simulink library "vmc"  (R2021b)
settings: Solver=VariableStepAuto  StartTime=0.0  StopTime=10.0  RelTol=1e-3
undefined symbols (not defined in the file or in its folder): AVMC_ACCDeltaTqIGain_X_kph, AVMC_ACCDeltaTqIGain_Y_mps2, AVMC_ACCDeltaTqIGainP2_X_kph, AVMC_ACCDeltaTqIGainP2_Y_mps2, AVMC_ACCDeltaTqPGain_X_kph, AVMC_ACCDeltaTqPGain_Y_kph, AVMC_ACCDeltaTqPGainP2_X_kph, AVMC_ACCDeltaTqPGainP2_Y_kph, AVMC_ACCLongSteadyCtrl_X_kph, AVMC_CCAccelCMD_X_kph, AVMC_CCAccelCMD_Y_kph, AVMC_CCDeltaTqIGain_X_kph, AVMC_CCDeltaTqIGain_Y_mps2, AVMC_CCDeltaTqPGain_X_kph, AVMC_CCDeltaTqPGain_Y_kph, AVMC_CCLongSteadyCtrl_X_kph, AVMC_DISCDeltaTqIGainP2_X_kph, AVMC_DISCDeltaTqIGainP2_Y_mps2, AVMC_ESCRegenOut_X_kph, AVMC_ESCRegenOut_Y_Deg, AVMC_ESCRegenOutEnSpd_X_Deg, AVMC_LatESCRegenOut_X_kph, AVMC_LatESCRegenOut_Y_Deg, AVMC_LongAccDeadZone_X_kph, AVMC_LongAccDeadZoneP2_X_kph, AVMC_LongAccFiltTs_X_Gps, AVMC_LongAccFiltTsP2_X_Gps, AVMC_MCPresBaseTq_X_bar, AVMC_MSAAccelCMD_X_kph, AVMC_MSAAccelCMD_Y_kph, AVMC_MSADeltaTqIGain_X_kph, AVMC_MSADeltaTqIGain_Y_mps2, AVMC_MSADeltaTqPGain_X_kph, AVMC_MSADeltaTqPGain_Y_kph, AVMC_MSALongSteadyCtrl_X_kph, AVMC_MSAPedalOvrd_X_kph, AVMC_MSASpdBand_X_kph, AVMC_OPDDisSlideRate_X_Deg, AVMC_RDCDetectTime_X_kph, AVMC_RDCDetectTime_Y_pct, AVMC_RDCEnSlideRate_X_Deg, AVMC_StESCYaw_X_kph, AVMC_StESCYaw_Y_Deg, AVMC_StESCYawCom_X_kph, AVMC_StESCYawCom_Y_Gps, AVMC_TMSpdBaseTq_X_rpm, C_TASK_10MS_S, C_TASK_5MS_S, DEG2RAD, Discrete, ENUM_ADASACCSTA_ACTIVE, ENUM_ADASACCSTA_OVERRIDE, ENUM_ADASACCSTA_STANDBY, ENUM_ADASMSASTA_ACTIVE, ENUM_ADASMSASTA_ERROR, ENUM_ADASMSASTA_OFF, ENUM_ADASMSASTA_OVERSPEED, ENUM_ADASMSASTA_STANDBY, ENUM_ADASMSASTA_UNDERSPEED, ENUM_ADASMSASTA_UNLIMIT ... (+254)
libraries: hcu_lib x57, simulink x49, ctrlSharedLib x6, simulink_extras x1
(part 3 of 9)

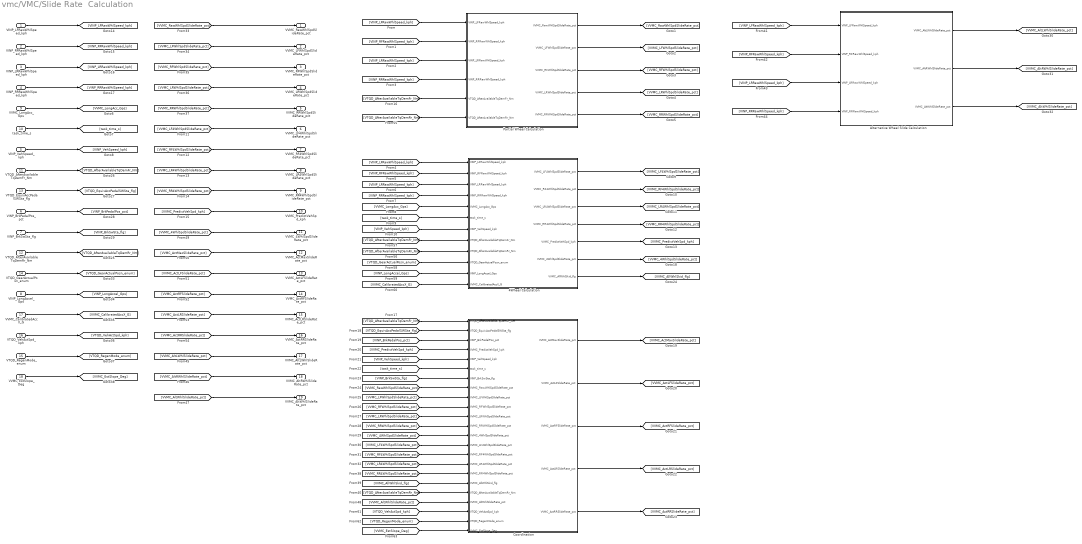
== system vmc/VMC/Slide Rate  Calculation ==
  VINP_LFRawWhlSpeed_kph : Inport
  VINP_RFRawWhlSpeed_kph : Inport  Port=2
  VINP_LRRawWhlSpeed_kph : Inport  Port=3
  VINP_RRRawWhlSpeed_kph : Inport  Port=4
  VINP_VehSpeed_kph : Inport  Port=5
  VINP_BrkPedalPos_pct : Inport  Port=6
  VINP_BrkSwSta_flg : Inport  Port=7
  VINP_LongAccel_Gps : Inport  Port=8
  VVMC_LongAcc_Gps : Inport  Port=9
  task_time_s : Inport  Port=10
  VTQD_AfterAvailableTqDemFr_Nm : Inport  Port=11
  VTQD_AfterAvailableTqDemRr_Nm : Inport  Port=12
  VTQD_EquivAccPedalSWSta_flg : Inport  Port=13
  VTQD_GearActualPosn_enum : Inport  Port=14
  VTQD_RegenMode_enum : Inport  Port=15
  VTQD_VehActSpd_kph : Inport  Port=16
  VVMC_CalibratedAccX_G : Inport  Port=17
  VVMC_EstSlope_Deg : Inport  Port=18
  4Wheel Calculation : Subsystem
  Alternative Wheel Slide Calculation : Subsystem
  Coordination : Subsystem
  Partial Wheel Calculation : Subsystem
  VVMC_RawWhlSpdSlideRate_pct : Outport
  VVMC_LFWhlSpdSlideRate_pct : Outport  Port=2
  VVMC_RFWhlSpdSlideRate_pct : Outport  Port=3
  VVMC_LRWhlSpdSlideRate_pct : Outport  Port=4
  VVMC_RRWhlSpdSlideRate_pct : Outport  Port=5
  VVMC_LF4WhlSpdSlideRate_pct : Outport  Port=6
  VVMC_RF4WhlSpdSlideRate_pct : Outport  Port=7
  VVMC_LR4WhlSpdSlideRate_pct : Outport  Port=8
  VVMC_RR4WhlSpdSlideRate_pct : Outport  Port=9
  VVMC_PredictVehSpd_kph : Outport  Port=10
  VVMC_4WhlSpdSlideRate_pct : Outport  Port=11
  VVMC_ActMaxSlideRate_pct : Outport  Port=12
  VVMC_ActLFSlideRate_pct : Outport  Port=13
  VVMC_ActRFSlideRate_pct : Outport  Port=14
  VVMC_ActLRSlideRate_pct : Outport  Port=15
  VVMC_ActRRSlideRate_pct : Outport  Port=16
  VVMC_AltLWhlSlideRate_pct : Outport  Port=17
  VVMC_AltRWhlSlideRate_pct : Outport  Port=18
  VVMC_AltWhlSlideRate_pct : Outport  Port=19
  wires:
  VINP_BrkSwSta_flg/1 -> [VINP_BrkSwSta_flg]
  VTQD_AfterAvailableTqDemFr_Nm/1 -> [VTQD_AfterAvailableTqDemFr_Nm]
  [VVMC_RF4WhlSpdSlideRate_pct] -> VVMC_RF4WhlSpdSlideRate_pct/1
  [VVMC_ActRRSlideRate_pct] -> VVMC_ActRRSlideRate_pct/1
  VTQD_EquivAccPedalSWSta_flg/1 -> [VTQD_EquivAccPedalSWSta_flg]
  [VVMC_LFWhlSpdSlideRate_pct] -> VVMC_LFWhlSpdSlideRate_pct/1
  VINP_BrkPedalPos_pct/1 -> [VINP_BrkPedalPos_pct]
  [VVMC_RRWhlSpdSlideRate_pct] -> VVMC_RRWhlSpdSlideRate_pct/1
  task_time_s/1 -> [task_time_s]
  VINP_RRRawWhlSpeed_kph/1 -> [VINP_RRRawWhlSpeed_kph]
  [VVMC_ActMaxSlideRate_pct] -> VVMC_ActMaxSlideRate_pct/1
  [VVMC_RFWhlSpdSlideRate_pct] -> VVMC_RFWhlSpdSlideRate_pct/1
  [VVMC_LR4WhlSpdSlideRate_pct] -> VVMC_LR4WhlSpdSlideRate_pct/1
  [VVMC_ActRFSlideRate_pct] -> VVMC_ActRFSlideRate_pct/1
  [VVMC_RR4WhlSpdSlideRate_pct] -> VVMC_RR4WhlSpdSlideRate_pct/1
  VINP_RFRawWhlSpeed_kph/1 -> [VINP_RFRawWhlSpeed_kph]
  VINP_VehSpeed_kph/1 -> [VINP_VehSpeed_kph]
  [VVMC_ActLRSlideRate_pct] -> VVMC_ActLRSlideRate_pct/1
  [VVMC_PredictVehSpd_kph] -> VVMC_PredictVehSpd_kph/1
  VINP_LRRawWhlSpeed_kph/1 -> [VINP_LRRawWhlSpeed_kph]
  [VVMC_LF4WhlSpdSlideRate_pct] -> VVMC_LF4WhlSpdSlideRate_pct/1
  [VVMC_RawWhlSpdSlideRate_pct] -> VVMC_RawWhlSpdSlideRate_pct/1
  VINP_LFRawWhlSpeed_kph/1 -> [VINP_LFRawWhlSpeed_kph]
  [VVMC_LRWhlSpdSlideRate_pct] -> VVMC_LRWhlSpdSlideRate_pct/1
  [VVMC_ActLFSlideRate_pct] -> VVMC_ActLFSlideRate_pct/1
  [VVMC_4WhlSpdSlideRate_pct] -> VVMC_4WhlSpdSlideRate_pct/1
  VVMC_LongAcc_Gps/1 -> [VVMC_LongAcc_Gps]
  VTQD_AfterAvailableTqDemRr_Nm/1 -> [VTQD_AfterAvailableTqDemRr_Nm]
  [VINP_LFRawWhlSpeed_kph] -> Alternative Wheel Slide Calculation/1(VINP_LFRawWhlSpeed_kph)
  [VINP_RFRawWhlSpeed_kph] -> Alternative Wheel Slide Calculation/2(VINP_RFRawWhlSpeed_kph)
  [VINP_LRRawWhlSpeed_kph] -> Alternative Wheel Slide Calculation/3(VINP_LRRawWhlSpeed_kph)
  [VINP_RRRawWhlSpeed_kph] -> Alternative Wheel Slide Calculation/4(VINP_RRRawWhlSpeed_kph)
  Alternative Wheel Slide Calculation/1(VVMC_AltLWhlSlideRate_pct) -> [VVMC_AltLWhlSlideRate_pct]
  Alternative Wheel Slide Calculation/2(VVMC_AltRWhlSlideRate_pct) -> [VVMC_AltRWhlSlideRate_pct]
  Alternative Wheel Slide Calculation/3(VVMC_AltWhlSlideRate_pct) -> [VVMC_AltWhlSlideRate_pct]
  [VVMC_AltLWhlSlideRate_pct] -> VVMC_AltLWhlSlideRate_pct/1
  [VVMC_AltRWhlSlideRate_pct] -> VVMC_AltRWhlSlideRate_pct/1
  [VVMC_AltWhlSlideRate_pct] -> VVMC_AltWhlSlideRate_pct/1
  Partial Wheel Calculation/2(VVMC_LFWhlSpdSlideRate_pct) -> [VVMC_LFWhlSpdSlideRate_pct]
  Partial Wheel Calculation/5(VVMC_RRWhlSpdSlideRate_pct) -> [VVMC_RRWhlSpdSlideRate_pct]
  Partial Wheel Calculation/3(VVMC_RFWhlSpdSlideRate_pct) -> [VVMC_RFWhlSpdSlideRate_pct]
  Partial Wheel Calculation/1(VVMC_RawWhlSpdSlideRate_pct) -> [VVMC_RawWhlSpdSlideRate_pct]
  [VINP_RFRawWhlSpeed_kph] -> Partial Wheel Calculation/2(VINP_RFRawWhlSpeed_kph)
  [VINP_LRRawWhlSpeed_kph] -> Partial Wheel Calculation/3(VINP_LRRawWhlSpeed_kph)
  [VTQD_AfterAvailableTqDemFr_Nm] -> Partial Wheel Calculation/5(VTQD_AfterAvailableTqDemFr_Nm)
  [VINP_LFRawWhlSpeed_kph] -> Partial Wheel Calculation/1(VINP_LFRawWhlSpeed_kph)
  [VINP_RRRawWhlSpeed_kph] -> Partial Wheel Calculation/4(VINP_RRRawWhlSpeed_kph)
  [VTQD_AfterAvailableTqDemRr_Nm] -> Partial Wheel Calculation/6(VTQD_AfterAvailableTqDemRr_Nm)
  Partial Wheel Calculation/4(VVMC_LRWhlSpdSlideRate_pct) -> [VVMC_LRWhlSpdSlideRate_pct]
  4Wheel Calculation/3(VVMC_LR4WhlSpdSlideRate_pct) -> [VVMC_LR4WhlSpdSlideRate_pct]
  [task_time_s] -> 4Wheel Calculation/6(task_time_s)
  4Wheel Calculation/1(VVMC_LF4WhlSpdSlideRate_pct) -> [VVMC_LF4WhlSpdSlideRate_pct]
  4Wheel Calculation/7(VVMC_AllWhlSkid_flg) -> [VVMC_AllWhlSkid_flg]
  [VVMC_LongAcc_Gps] -> 4Wheel Calculation/5(VVMC_LongAcc_Gps)
  4Wheel Calculation/4(VVMC_RR4WhlSpdSlideRate_pct) -> [VVMC_RR4WhlSpdSlideRate_pct]
  [VTQD_AfterAvailableTqDemRr_Nm] -> 4Wheel Calculation/9(VTQD_AfterAvailableTqDemRr_Nm)
  [VTQD_AfterAvailableTqDemFr_Nm] -> 4Wheel Calculation/8(VTQD_AfterAvailableTqDemFr_Nm)
  [VINP_VehSpeed_kph] -> 4Wheel Calculation/7(VINP_VehSpeed_kph)
  4Wheel Calculation/5(VVMC_PredictVehSpd_kph) -> [VVMC_PredictVehSpd_kph]
  [VINP_LRRawWhlSpeed_kph] -> 4Wheel Calculation/3(VINP_LRRawWhlSpeed_kph)
  [VINP_RRRawWhlSpeed_kph] -> 4Wheel Calculation/4(VINP_RRRawWhlSpeed_kph)
  [VINP_LFRawWhlSpeed_kph] -> 4Wheel Calculation/1(VINP_LFRawWhlSpeed_kph)
  [VINP_RFRawWhlSpeed_kph] -> 4Wheel Calculation/2(VINP_RFRawWhlSpeed_kph)
  4Wheel Calculation/2(VVMC_RF4WhlSpdSlideRate_pct) -> [VVMC_RF4WhlSpdSlideRate_pct]
  4Wheel Calculation/6(VVMC_4WhlSpdSlideRate_pct) -> [VVMC_4WhlSpdSlideRate_pct]
  [VVMC_LF4WhlSpdSlideRate_pct] -> Coordination/14(VVMC_LF4WhlSpdSlideRate_pct)
  [VVMC_RR4WhlSpdSlideRate_pct] -> Coordination/17(VVMC_RR4WhlSpdSlideRate_pct)
  [VVMC_LR4WhlSpdSlideRate_pct] -> Coordination/16(VVMC_LR4WhlSpdSlideRate_pct)
  [task_time_s] -> Coordination/6(task_time_s)
  [VVMC_LFWhlSpdSlideRate_pct] -> Coordination/9(VVMC_LFWhlSpdSlideRate_pct)
  [VTQD_AfterAvailableTqDemFr_Nm] -> Coordination/1(VTQD_AfterAvailableTqDemFr_Nm)
  [VVMC_AltWhlSlideRate_pct] -> Coordination/20(VVMC_AltWhlSlideRate_pct)
  [VVMC_RFWhlSpdSlideRate_pct] -> Coordination/10(VVMC_RFWhlSpdSlideRate_pct)
  [VTQD_EquivAccPedalSWSta_flg] -> Coordination/2(VTQD_EquivAccPedalSWSta_flg)
  [VVMC_AllWhlSkid_flg] -> Coordination/18(VVMC_AllWhlSkid_flg)
  [VVMC_4WhlSpdSlideRate_pct] -> Coordination/13(VVMC_4WhlSpdSlideRate_pct)
  [VINP_VehSpeed_kph] -> Coordination/5(VINP_VehSpeed_kph)
  Coordination/3(VVMC_ActRFSlideRate_pct) -> [VVMC_ActRFSlideRate_pct]
  [VVMC_RawWhlSpdSlideRate_pct] -> Coordination/8(VVMC_RawWhlSpdSlideRate_pct)
  [VTQD_AfterAvailableTqDemRr_Nm] -> Coordination/19(VTQD_AfterAvailableTqDemRr_Nm)
  Coordination/4(VVMC_ActLRSlideRate_pct) -> [VVMC_ActLRSlideRate_pct]
  [VVMC_PredictVehSpd_kph] -> Coordination/4(VVMC_PredictVehSpd_kph)
  [VINP_BrkSwSta_flg] -> Coordination/7(VINP_BrkSwSta_flg)
  [VVMC_LRWhlSpdSlideRate_pct] -> Coordination/11(VVMC_LRWhlSpdSlideRate_pct)
  [VVMC_RRWhlSpdSlideRate_pct] -> Coordination/12(VVMC_RRWhlSpdSlideRate_pct)
  [VINP_BrkPedalPos_pct] -> Coordination/3(VINP_BrkPedalPos_pct)
  Coordination/1(VVMC_ActMaxSlideRate_pct) -> [VVMC_ActMaxSlideRate_pct]
  Coordination/5(VVMC_ActRRSlideRate_pct) -> [VVMC_ActRRSlideRate_pct]
  Coordination/2(VVMC_ActLFSlideRate_pct) -> [VVMC_ActLFSlideRate_pct]
  [VVMC_RF4WhlSpdSlideRate_pct] -> Coordination/15(VVMC_RF4WhlSpdSlideRate_pct)
  [VTQD_GearActualPosn_enum] -> 4Wheel Calculation/10(VTQD_GearActualPosn_enum)
  VTQD_GearActualPosn_enum/1 -> [VTQD_GearActualPosn_enum]
  VINP_LongAccel_Gps/1 -> [VINP_LongAccel_Gps]
  [VINP_LongAccel_Gps] -> 4Wheel Calculation/11(VINP_LongAccel_Gps)
  [VVMC_CalibratedAccX_G] -> 4Wheel Calculation/12(VVMC_CalibratedAccX_G)
  VVMC_CalibratedAccX_G/1 -> [VVMC_CalibratedAccX_G]
  VVMC_EstSlope_Deg/1 -> [VVMC_EstSlope_Deg]
  VTQD_RegenMode_enum/1 -> [VTQD_RegenMode_enum]
  VTQD_VehActSpd_kph/1 -> [VTQD_VehActSpd_kph]
  [VTQD_RegenMode_enum] -> Coordination/22(VTQD_RegenMode_enum)
  [VTQD_VehActSpd_kph] -> Coordination/21(VTQD_VehActSpd_kph)
  [VVMC_EstSlope_Deg] -> Coordination/23(VVMC_EstSlope_Deg)

== system vmc/VMC/Subsystem1 ==
  note: TRUE
  VINP_VehSpeed_kph : Inport
  VINP_ACCRequiredAccel_mps2 : Inport  Port=2
  VINP_ACCVehHoldReq_flg : Inport  Port=3
  VINP_ACCObjRelSpd_mps : Inport  Port=4
  VINP_ACCObjDist_m : Inport  Port=5
  VINP_TimeGapLevel_enum : Inport  Port=6
  VTQD_FrEDUAvailBrkRgnTq_Nm : Inport  Port=7
  VTQD_RrEDUAvailBrkRgnTq_Nm : Inport  Port=8
  VINP_METERKPHCalcu_kph : Inport  Port=9
  0 : Constant  Value=KVMC_AllowSetSpdOvrd_flg
  1 : Constant  Value=KVMC_AllowSetSpdOvrdVal_flg
  10kph1 : Constant  Value=KVMC_AllowSetSpdSpd_kph
  20m : Constant  Value=KVMC_AllowSetSpdDist_m
  2m : Constant  Value=KVMC_NotAllowSetSpdDist_m
  AND : Logic  AllPortsSameDT=off  OutDataTypeStr=boolean
  AND2 : Logic  Inputs=3  AllPortsSameDT=off  OutDataTypeStr=boolean
  Add : Sum
  Cast To Single : DataTypeConversion  OutDataTypeStr=single
  Constant1 : Constant  Value=KPH2MPS
  Constant10 : Constant  Value=ENUM_TIMEGAPLEVEL_LEVEL1
  Constant11 : Constant  Value=ENUM_TIMEGAPLEVEL_LEVEL2
  Constant12 : Constant  Value=ENUM_TIMEGAPLEVEL_LEVEL3
  Constant13 : Constant  Value=ENUM_TIMEGAPLEVEL_LEVEL4
  Constant14 : Constant  Value=KVMC_TimeGapBandLv2_s
  Constant15 : Constant  Value=KVMC_TimeGapBandLv3_s
  Constant16 : Constant  Value=KVMC_TimeGapBandLv4_s
  Constant17 : Constant  Value=TRUE
  Constant18 : Constant  Value=FALSE
  Constant19 : Constant  Value=ZERO_FLOAT
  Constant2 : Constant  Value=KVMC_TimeGapBandLv1_s
  Constant47 : Constant  Value=KVMC_TimeGapMax_s
  Constant48 : Constant  Value=ZERO_FLOAT
  Constant5 : Constant  Value=ZERO_FLOAT
  Constant6 : Constant  Value=KVMC_PosAccelHoldDelaySW_flg
  Constant7 : Constant  Value=KVMC_TimeGapMax_s
  Constant8 : Constant  Value=TRUE
  Constant9 : Constant  Value=FALSE
  Detect Increase1 : simulink/Logic and Bit Operations/Detect Increase  vinit=0.0  OutDataTypeStr=boolean
  Merge1 : Merge
  NOT1 : Logic  Operator=NOT  AllPortsSameDT=off  OutDataTypeStr=boolean
  OR : Logic  Operator=OR  AllPortsSameDT=off  OutDataTypeStr=boolean
  Relational Operator : RelationalOperator  Operator=<=  OutDataTypeStr=boolean  RndMeth=Simplest
  Relational Operator1 : RelationalOperator  Operator=>  OutDataTypeStr=boolean  RndMeth=Simplest
  Relational Operator2 : RelationalOperator  OutDataTypeStr=boolean  RndMeth=Simplest
  Relational Operator3 : RelationalOperator  OutDataTypeStr=boolean  RndMeth=Simplest
  Saturation Dynamic2 : simulink/Discontinuities/Saturation Dynamic  OutMin=[]  OutMax=[]  OutDataTypeStr=Inherit: Same as second input  OutDataType=fixdt(1, 16)  OutScaling=2^-10  DoSatur=off
  Switch : Switch  Criteria=u2 > Threshold
  TimeGapJudgement : Stateflow chart  TreatAsAtomicUnit=on
  Triggered Subsystem2 : Subsystem  TreatAsAtomicUnit=on
  Triggered Subsystem3 : Subsystem  TreatAsAtomicUnit=on
  Unit Delay3 : UnitDelay  SampleTime=-1  HasFrameUpgradeWarning=on
  VVMC_AccelTurnHold_flg : Outport
  VVMC_TotalAvailBrkRgnTq_Nm : Outport  Port=2
  VVMC_TimeGapJudge_flag : Outport  Port=3
  VVMC_AllowSetSpd_flg : Outport  Port=4
  wires:
  AND2/1 -> Triggered Subsystem2/Trigger
  Constant9/1 -> Triggered Subsystem3/1(In1)
  [VINP_ACCVehHoldReq_flg] -> NOT1/1
  NOT1/1 -> Triggered Subsystem3/Trigger
  Constant8/1 -> Triggered Subsystem2/1(In1)
  Triggered Subsystem3/1(Out1) -> Merge1/2
  Triggered Subsystem2/1(Out1) -> Merge1/1
  Merge1/1 -> [VVMC_AccelTurnHold_flg]
  Relational Operator2/1 -> AND2/1
  Constant5/1 -> Relational Operator2/2
  Detect Increase1/1 -> AND2/2
  [VINP_ACCRequiredAccel_mps2] -> Unit Delay3/1
  Unit Delay3/1 -> Relational Operator2/1
  Constant6/1 -> AND2/3
  [VINP_ACCVehHoldReq_flg] -> Detect Increase1/1
  VINP_ACCRequiredAccel_mps2/1 -> [VINP_ACCRequiredAccel_mps2]
  VINP_ACCVehHoldReq_flg/1 -> [VINP_ACCVehHoldReq_flg]
  [VVMC_AccelTurnHold_flg] -> VVMC_AccelTurnHold_flg/1
  [VTQD_RrEDUAvailBrkRgnTq_Nm] -> Add/2
  Add/1 -> [VVMC_TotalAvailBrkRgnTq_Nm]
  [VTQD_FrEDUAvailBrkRgnTq_Nm] -> Add/1
  VTQD_RrEDUAvailBrkRgnTq_Nm/1 -> [VTQD_RrEDUAvailBrkRgnTq_Nm]
  VTQD_FrEDUAvailBrkRgnTq_Nm/1 -> [VTQD_FrEDUAvailBrkRgnTq_Nm]
  [VVMC_TotalAvailBrkRgnTq_Nm] -> VVMC_TotalAvailBrkRgnTq_Nm/1
  Constant15/1 -> TimeGapJudgement/11(KVMC_TimeGapBandLv3_s)
  Constant18/1 -> TimeGapJudgement/15(FALSE)
  [VINP_VehSpeed_kph] -> TimeGapJudgement/3(VINP_VehSpeed_kph)
  Cast To Single/1 -> Saturation Dynamic2/2
  Constant47/1 -> Saturation Dynamic2/1
  [VINP_ACCObjRelSpd_mps] -> TimeGapJudgement/1(VINP_ACCObjRelSpd_mps)
  Saturation Dynamic2/1 -> [VVMC_TimeGapCalcu_s]  "VVMC_TimeGapCalcu_s"
  Constant2/1 -> TimeGapJudgement/7(KVMC_TimeGapBandLv1_s)
  TimeGapJudgement/2(VVMC_TimeGapCalcu_s) -> Cast To Single/1
  Constant48/1 -> Saturation Dynamic2/3
  Constant17/1 -> TimeGapJudgement/14(TRUE)
  Constant1/1 -> TimeGapJudgement/4(KPH2MPS)
  Constant11/1 -> TimeGapJudgement/8(ENUM_TIMEGAPLEVEL_LEVEL2)
  Constant19/1 -> TimeGapJudgement/16(ZERO_FLOAT)
  Constant16/1 -> TimeGapJudgement/13(KVMC_TimeGapBandLv4_s)
  Constant12/1 -> TimeGapJudgement/10(ENUM_TIMEGAPLEVEL_LEVEL3)
  [VINP_ACCObjDist_m] -> TimeGapJudgement/2(VINP_ACCObjDist_m)
  Constant10/1 -> TimeGapJudgement/6(ENUM_TIMEGAPLEVEL_LEVEL1)
  TimeGapJudgement/1(VVMC_TimeGapJudge_flag) -> [VVMC_TimeGapJudge_flag]  "VVMC_TimeGapJudge_flag"
  [VINP_TimeGapLevel_enum] -> TimeGapJudgement/5(VINP_TimeGapLevel_enum)
  Constant14/1 -> TimeGapJudgement/9(KVMC_TimeGapBandLv2_s)
  Constant7/1 -> TimeGapJudgement/17(KVMC_TimeGapMax_s)
  Constant13/1 -> TimeGapJudgement/12(ENUM_TIMEGAPLEVEL_LEVEL4)
  VINP_ACCObjRelSpd_mps/1 -> [VINP_ACCObjRelSpd_mps]
  VINP_ACCObjDist_m/1 -> [VINP_ACCObjDist_m]
  VINP_VehSpeed_kph/1 -> [VINP_VehSpeed_kph]
  VINP_TimeGapLevel_enum/1 -> [VINP_TimeGapLevel_enum]
  [VVMC_TimeGapJudge_flag] -> VVMC_TimeGapJudge_flag/1
  Relational Operator3/1 -> OR/2
  AND/1 -> OR/1
  OR/1 -> Switch/3
  [VINP_METERKPHCalcu_kph] -> Relational Operator3/1
  0/1 -> Switch/2
  1/1 -> Switch/1
  Relational Operator1/1 -> AND/2
  10kph1/1 -> Relational Operator3/2
  Switch/1 -> [VVMC_AllowSetSpd_flg]  "VVMC_AllowSetSpd_flg"
  Relational Operator/1 -> AND/1
  [VINP_ACCObjDist_m] -> Relational Operator/1, Relational Operator1/1
  2m/1 -> Relational Operator1/2
  20m/1 -> Relational Operator/2
  [VVMC_AllowSetSpd_flg] -> VVMC_AllowSetSpd_flg/1
  VINP_METERKPHCalcu_kph/1 -> [VINP_METERKPHCalcu_kph]

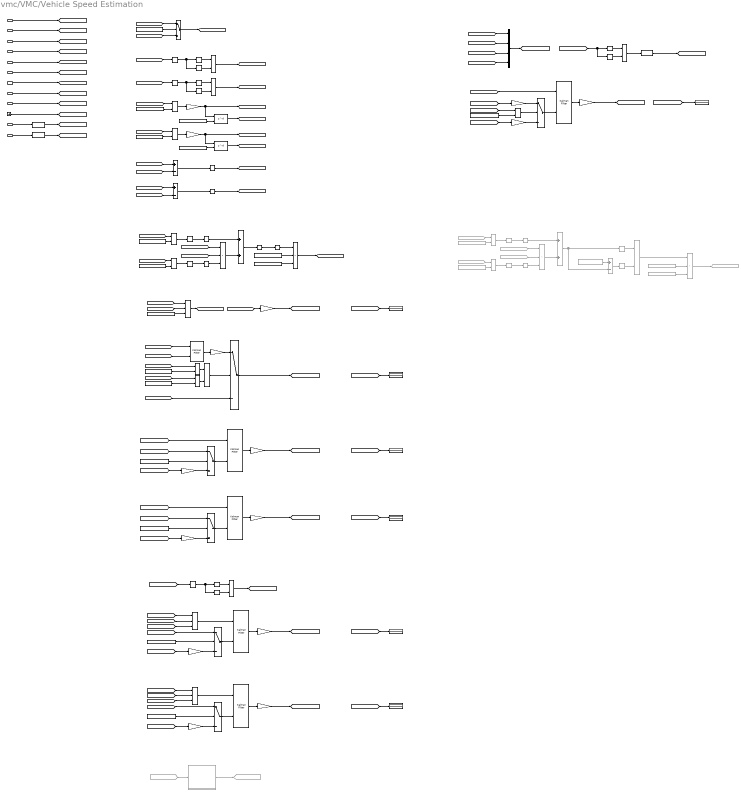
== system vmc/VMC/Vehicle Speed Estimation ==
  note: GPS
  note: RawWhl
  VINP_LFRawWhlSpeed_kph : Inport
  VINP_RFRawWhlSpeed_kph : Inport  Port=2
  VINP_LRRawWhlSpeed_kph : Inport  Port=3
  VINP_RRRawWhlSpeed_kph : Inport  Port=4
  VINP_VehSpeed_kph : Inport  Port=5
  VINP_LongAccel_Gps : Inport  Port=6
  VINP_GPSLAT_sec : Inport  Port=7
  VINP_GPSLONG_sec : Inport  Port=8
  VVMC_LongAcc_Gps : Inport  Port=9
  task_time_s : Inport  Port=10
  VTQD_GearActualPosn_enum : Inport  Port=11
  Abs : Abs
  Abs1 : Abs
  Asin : Trigonometry  Operator=asin
  Atan1 : Trigonometry  Commented=on  Operator=atan2
  Constant : Constant  Value=1000000  OutDataTypeStr=single
  Constant1 : Constant  Value=1000000  OutDataTypeStr=single
  Constant{10,14,17..18,20} (5 alike) : Constant  Value=KVMC_PreVehSpdCalSW_flg
  Constant11 : Constant  Commented=on  Value=ONE_FLOAT  OutDataTypeStr=single
  Constant12 : Constant  Commented=on  Value=2  OutDataTypeStr=single
  Constant13 : Constant  Commented=on  Value=6371004  OutDataTypeStr=single
  Constant15 : Constant  Value=KVMC_GPSRollAveNum_c  OutDataTypeStr=single
  Constant16 : Constant  Value=KVMC_GPSRollAveNum_c  OutDataTypeStr=single
  Constant2 : Constant  Commented=on  Value=2  OutDataTypeStr=single
  Constant3 : Constant  Value=KVMC_4WheelLongAccSW_flg
  Constant4 : Constant  Commented=on  Value=2  OutDataTypeStr=single
  Constant46 : Constant  Value=ENUM_GEARACTUALPOSN_D
  Constant47 : Constant  Value=ENUM_GEARACTUALPOSN_R
  Constant5 : Constant  Value=2  OutDataTypeStr=single
  Constant6 : Constant  Value=2  OutDataTypeStr=single
  Constant7 : Constant  Value=KVMC_GPSRollAveNum_c  OutDataTypeStr=single
  Constant8 : Constant  Value=2  OutDataTypeStr=single
  Constant9 : Constant  Value=KVMC_GPSEarthRadius_c  OutDataTypeStr=single
  Data Type Conversion : DataTypeConversion  OutDataTypeStr=single
  Data Type Conversion1 : DataTypeConversion  OutDataTypeStr=single
  Data Type Conversion2 : DataTypeConversion  OutDataTypeStr=single
  Delay : Delay  DelayLengthSource=Input port  DelayLength=50  DelayLengthUpperLimit=5000
      settings: InputPortMap=u0,p1
  Delay1 : Delay  DelayLengthSource=Input port  DelayLength=50  DelayLengthUpperLimit=5000
      settings: InputPortMap=u0,p1
  Display{,1..6} (7 alike) : Display
  Divide{,1..3} (4 alike) : Product  Inputs=*/
  Divide10 : Product  Commented=on  Inputs=***
  Divide11 : Product  Inputs=**/
  Divide12 : Product  Inputs=**/
  Divide4 : Product  Inputs=***
  Divide5 : Product  Inputs=***
  Divide6 : Product  Inputs=*//
  Divide7 : Product  Commented=on  Inputs=*/
  Divide8 : Product  Commented=on  Inputs=*/
  Divide9 : Product  Commented=on  Inputs=***
  Equal : RelationalOperator  Operator===  OutDataTypeStr=boolean  RndMeth=Simplest
  Equal1 : RelationalOperator  Operator===  OutDataTypeStr=boolean  RndMeth=Simplest
  From13 : From  Commented=on  GotoTag=VVMC_GPSLATDelay_rad
  From15 : From  Commented=on  GotoTag=VVMC_GPSLATDelta_rad
  From32 : From  Commented=on  GotoTag=VVMC_GPSLONGDelta_rad
  From50 : From  Commented=on  GotoTag=task_time_s
  From8 : From  Commented=on  GotoTag=VVMC_GPSLAT_rad
  Gain : Gain  Gain=DEG2RAD  OutDataTypeStr=single
  Gain1 : Gain  Gain=DEG2RAD  OutDataTypeStr=single
  Gain{5,7..8,10,12,14} (6 alike) : Gain  Gain=KPH2MPS  OutDataTypeStr=single
  Gain{2..4,6,9,11,13} (7 alike) : Gain  Gain=MPS2KPH  OutDataTypeStr=single
  Goto25 : Goto  Commented=on  GotoTag=VVMC_GPSDisDelta_m
  Goto31 : Goto  Commented=on  GotoTag=trig_KF_10s
  Ground : Ground
  Kalman Filter1 : ctrlSharedLib/Kalman Filter  TimeDomain=Discrete-Time  UseCurrentEstimator=on  ModelSource=Individual A, B, C, D matrices  ModelSourceVariable=ss(0.95,1,1,0,1)  A=1  B=C_TASK_5MS_S  C=1  D=0  NumberOfStates=1  NumberOfInputs=1  NumberOfOutputs=1  InitialEstimateSource=Dialog  X0=0  P0=10  UseK=off  UseGH=off  NumberOfProcessNoiseInputs=1  G=1  TimeInvariantG=on  H=0  TimeInvariantH=on  Q=0.01  TimeInvariantQ=on  R=0.03  TimeInvariantR=on  N=0  TimeInvariantN=on  AddInputPort=on  AddEnablePort=off  OutputEstimatedY=off  OutputP=off  Ts=-1
  Kalman Filter2 : ctrlSharedLib/Kalman Filter  TimeDomain=Discrete-Time  UseCurrentEstimator=on  ModelSource=Individual A, B, C, D matrices  ModelSourceVariable=ss(0.95,1,1,0,1)  A=1  B=C_TASK_5MS_S  C=1  D=0  NumberOfStates=1  NumberOfInputs=1  NumberOfOutputs=1  InitialEstimateSource=Dialog  X0=0  P0=10  UseK=off  UseGH=off  NumberOfProcessNoiseInputs=1  G=1  TimeInvariantG=on  H=0  TimeInvariantH=on  Q=0.03  TimeInvariantQ=on  R=0.01  TimeInvariantR=on  N=0  TimeInvariantN=on  AddInputPort=on  AddEnablePort=off  OutputEstimatedY=off  OutputP=off  Ts=-1
  Kalman Filter3 : ctrlSharedLib/Kalman Filter  TimeDomain=Discrete-Time  UseCurrentEstimator=on  ModelSource=Individual A, B, C, D matrices  ModelSourceVariable=ss(0.95,1,1,0,1)  A=1  B=C_TASK_5MS_S  C=1  D=0  NumberOfStates=1  NumberOfInputs=1  NumberOfOutputs=1  InitialEstimateSource=Dialog  X0=0  P0=10  UseK=off  UseGH=off  NumberOfProcessNoiseInputs=1  G=1  TimeInvariantG=on  H=0  TimeInvariantH=on  Q=0.03  TimeInvariantQ=on  R=0.01  TimeInvariantR=on  N=0  TimeInvariantN=on  AddInputPort=on  AddEnablePort=off  OutputEstimatedY=off  OutputP=off  Ts=-1
  Kalman Filter4 : ctrlSharedLib/Kalman Filter  TimeDomain=Discrete-Time  UseCurrentEstimator=on  ModelSource=Individual A, B, C, D matrices  ModelSourceVariable=ss(0.95,1,1,0,1)  A=1  B=C_TASK_5MS_S  C=1  D=0  NumberOfStates=1  NumberOfInputs=1  NumberOfOutputs=1  InitialEstimateSource=Dialog  X0=0  P0=10  UseK=off  UseGH=off  NumberOfProcessNoiseInputs=1  G=1  TimeInvariantG=on  H=0  TimeInvariantH=on  Q=0.01  TimeInvariantQ=on  R=0.03  TimeInvariantR=on  N=0  TimeInvariantN=on  AddInputPort=on  AddEnablePort=off  OutputEstimatedY=off  OutputP=off  Ts=-1
  Kalman Filter5 : ctrlSharedLib/Kalman Filter  TimeDomain=Discrete-Time  UseCurrentEstimator=on  ModelSource=Individual A, B, C, D matrices  ModelSourceVariable=ss(0.95,1,1,0,1)  A=1  B=C_TASK_5MS_S  C=1  D=0  NumberOfStates=1  NumberOfInputs=1  NumberOfOutputs=1  InitialEstimateSource=Dialog  X0=0  P0=10  UseK=off  UseGH=off  NumberOfProcessNoiseInputs=1  G=1  TimeInvariantG=on  H=0  TimeInvariantH=on  Q=0.01  TimeInvariantQ=on  R=0.03  TimeInvariantR=on  N=0  TimeInvariantN=on  AddInputPort=on  AddEnablePort=off  OutputEstimatedY=off  OutputP=off  Ts=-1
  Kalman Filter6 : ctrlSharedLib/Kalman Filter  TimeDomain=Discrete-Time  UseCurrentEstimator=on  ModelSource=Individual A, B, C, D matrices  ModelSourceVariable=ss(0.95,1,1,0,1)  A=1  B=C_TASK_5MS_S  C=1  D=0  NumberOfStates=1  NumberOfInputs=1  NumberOfOutputs=1  InitialEstimateSource=Dialog  X0=0  P0=10  UseK=off  UseGH=off  NumberOfProcessNoiseInputs=1  G=1  TimeInvariantG=on  H=0  TimeInvariantH=on  Q=0.03  TimeInvariantQ=on  R=0.01  TimeInvariantR=on  N=0  TimeInvariantN=on  AddInputPort=on  AddEnablePort=off  OutputEstimatedY=off  OutputP=off  Ts=-1
  Minus : Sum  Inputs=+-
  Minus1 : Sum  Inputs=+-
  Minus2 : Sum
  Minus4 : Sum  Commented=on
  Minus5 : Sum  Commented=on  Inputs=+-
  Mux : Mux
  OR : Logic  Operator=OR  AllPortsSameDT=off  OutDataTypeStr=boolean
  OR1 : Logic  Operator=OR  AllPortsSameDT=off  OutDataTypeStr=boolean
  Product{,1..3} (4 alike) : Product  Inputs=*/
  Scheduler : Stateflow chart  Commented=on  TreatAsAtomicUnit=on
  Sin : Trigonometry
  Sin1 : Trigonometry
  Sin2 : Trigonometry  Commented=on
  Sin3 : Trigonometry  Commented=on
  Sqrt : Sqrt  SaturateOnIntegerOverflow=on
  Sqrt2 : Sqrt  Commented=on  SaturateOnIntegerOverflow=on
  Sqrt3 : Sqrt  Commented=on  SaturateOnIntegerOverflow=on
  Square : Math  Operator=square  SaturateOnIntegerOverflow=on
  Square1 : Math  Operator=square  SaturateOnIntegerOverflow=on
  Square2 : Math  Commented=on  Operator=square  SaturateOnIntegerOverflow=on
  Square3 : Math  Commented=on  Operator=square  SaturateOnIntegerOverflow=on
  Sum of Elements{,1..3} (4 alike) : Sum  Inputs=+
  Switch{,1..5,10} (7 alike) : Switch  Criteria=u2 > Threshold
  Tapped Delay1 : simulink/Discrete/Tapped Delay  vinit=0.0  samptime=-1  NumDelays=2000  DelayOrder=Newest  includeCurrent=on
  Tapped Delay2 : simulink/Discrete/Tapped Delay  vinit=0.0  samptime=-1  NumDelays=1999  DelayOrder=Newest  includeCurrent=on
  Tapped Delay3 : simulink/Discrete/Tapped Delay  vinit=0.0  samptime=-1  NumDelays=2000  DelayOrder=Newest  includeCurrent=on
  Width{,1..3} (4 alike) : Width
  wires:
  task_time_s/1 -> [task_time_s]
  VINP_RRRawWhlSpeed_kph/1 -> [VINP_RRRawWhlSpeed_kph]
  VINP_RFRawWhlSpeed_kph/1 -> [VINP_RFRawWhlSpeed_kph]
  VINP_VehSpeed_kph/1 -> [VINP_VehSpeed_kph]
  VINP_LRRawWhlSpeed_kph/1 -> [VINP_LRRawWhlSpeed_kph]
  VINP_LFRawWhlSpeed_kph/1 -> [VINP_LFRawWhlSpeed_kph]
  VTQD_GearActualPosn_enum/1 -> [VTQD_GearActualPosn_enum]
  VINP_LongAccel_Gps/1 -> [VINP_LongAccel_Gps]
  [VTQD_GearActualPosn_enum] -> Equal1/1
  Constant47/1 -> Equal1/2
  Constant46/1 -> Equal/2
  Equal/1 -> OR/1
  [VINP_VehSpeed_kph] -> Switch10/3
  Switch10/1 -> [VVMC_EstVehSpd_kph]  "VVMC_EstVehSpd_kph"
  OR/1 -> Switch10/2
  Equal1/1 -> OR/2
  [VTQD_GearActualPosn_enum] -> Equal/1
  [VVMC_LongAcc4Whl_Gps] -> Kalman Filter1/1
  [VINP_LFRawWhlSpeed_kph] -> Mux/1
  [VINP_RRRawWhlSpeed_kph] -> Mux/4
  [VINP_LRRawWhlSpeed_kph] -> Mux/3
  [VINP_RFRawWhlSpeed_kph] -> Mux/2
  Mux/1 -> [VVMC_4WheelRawWhlSpeed_kph]
  Width/1 -> Product/2
  Sum of Elements/1 -> Product/1
  [VVMC_4WheelRawWhlSpeed_kph] -> Width/1, Sum of Elements/1
  [VVMC_GPSSpd_mps] -> Kalman Filter1/2
  Kalman Filter3/1 -> Gain4/1
  [VVMC_LongAcc4Whl_Gps] -> Kalman Filter3/1
  Ground/1 -> [VVMC_LFWhlSkid_flg]
  Product/1 -> Data Type Conversion/1
  Data Type Conversion/1 -> [VVMC_AvgRawWhlSpeed_kph]  "VVMC_AvgRawWhlSpeed_kph"
  [VVMC_EstVehSpd_kph] -> Display/1
  [VVMC_GPSLATRollAvg_sec] -> Divide/1
  Constant/1 -> Divide/2
  Constant1/1 -> Divide1/2
  [VVMC_GPSLONGRollAvg_sec] -> Divide1/1
  Delay/1 -> [VVMC_GPSLATDelay_rad]
  [VVMC_GPSLAT_rad] -> Minus/1
  Minus/1 -> Abs/1
  [VVMC_GPSLATDelay_rad] -> Minus/2
  Minus1/1 -> Abs1/1
  [VVMC_GPSLONG_rad] -> Minus1/1
  [VVMC_GPSLONGDelay_rad] -> Minus1/2
  Abs/1 -> [VVMC_GPSLATDelta_rad]
  Abs1/1 -> [VVMC_GPSLONGDelta_rad]
  [VVMC_GPSLATDelta_rad] -> Divide2/1
  Constant5/1 -> Divide2/2
  Divide2/1 -> Sin/1
  Sin/1 -> Square/1
  Constant6/1 -> Divide3/2
  [VVMC_GPSLONGDelta_rad] -> Divide3/1
  Divide3/1 -> Sin1/1
  Sin1/1 -> Square1/1
  Divide4/1 -> Minus2/2
  Square/1 -> Minus2/1
  [VVMC_GPSLATDelay_rad] -> Divide4/2
  [VVMC_GPSLAT_rad] -> Divide4/1
  Square1/1 -> Divide4/3
  Minus2/1 -> Sqrt/1
  Sqrt/1 -> Asin/1
  Asin/1 -> Divide5/1
  Constant8/1 -> Divide5/2
  Constant9/1 -> Divide5/3
  Divide5/1 -> [VVMC_GPSDeltaDis_m]
  Divide/1 -> Gain/1
  Gain/1 -> Delay/1, [VVMC_GPSLAT_rad]
  Divide1/1 -> Gain1/1
  [VINP_GPSLAT_sec] -> Tapped Delay1/1
  Width2/1 -> Product2/2
  Sum of Elements2/1 -> Product2/1
  Tapped Delay1/1 -> Sum of Elements2/1, Width2/1
  Product2/1 -> [VVMC_GPSLATRollAvg_sec]
  Product3/1 -> [VVMC_GPSLONGRollAvg_sec]
  Tapped Delay3/1 -> Width3/1, Sum of Elements3/1
  Sum of Elements3/1 -> Product3/1
  Width3/1 -> Product3/2
  [VINP_GPSLONG_sec] -> Tapped Delay3/1
  Kalman Filter1/1 -> Gain2/1
  Gain2/1 -> Switch10/1
  [VVMC_GPSSpd_mps] -> Gain3/1
  Gain3/1 -> [VVMC_GPSSpd_kph]  "VVMC_GPSSpd_kph"
  [VVMC_GPSSpd_kph] -> Display2/1
  Constant10/1 -> Switch2/2
  Switch2/1 -> Kalman Filter3/2
  [VVMC_GPSEstSpeed_kph] -> Display3/1
  Gain4/1 -> [VVMC_GPSEstSpeed_kph]  "VVMC_GPSEstSpeed_kph"
  Gain5/1 -> Switch2/3
  [VINP_VehSpeed_kph] -> Gain5/1
  [VVMC_GPSSpd_mps] -> Switch2/1
  Divide10/1 -> Goto25/1
  Constant13/1 -> Divide10/3
  Constant12/1 -> Divide10/2
  Atan1/1 -> Divide10/1
  Sqrt2/1 -> Atan1/1
  Sqrt3/1 -> Atan1/2
  Minus5/1 -> Sqrt3/1
  Constant11/1 -> Minus5/1
  Minus4/1 -> Sqrt2/1, Minus5/2
  Square3/1 -> Divide9/3
  From8/1 -> Divide9/1
  From13/1 -> Divide9/2
  Square2/1 -> Minus4/1
  Divide9/1 -> Minus4/2
  Sin3/1 -> Square3/1
  Divide8/1 -> Sin3/1
  From32/1 -> Divide8/1
  Constant4/1 -> Divide8/2
  Sin2/1 -> Square2/1
  Divide7/1 -> Sin2/1
  Constant2/1 -> Divide7/2
  From15/1 -> Divide7/1
  Constant7/1 -> Divide6/3
  [task_time_s] -> Divide6/2
  Divide6/1 -> [VVMC_GPSSpd_mps]
  [VVMC_GPSDeltaDis_m] -> Divide6/1
  Delay1/1 -> [VVMC_GPSLONGDelay_rad]
  [VINP_VehSpeed_kph] -> Gain7/1
  Gain7/1 -> Switch1/3
  Gain6/1 -> [VVMC_RawWhlEstSpeed_kph]  "VVMC_RawWhlEstSpeed_kph"
  [VVMC_RawWhlEstSpeed_kph] -> Display1/1
  Switch1/1 -> Kalman Filter2/2
  Constant14/1 -> OR1/2
  OR1/1 -> Switch1/2
  [VVMC_LFWhlSkid_flg] -> OR1/1
  [VVMC_LongAcc4Whl_Gps] -> Kalman Filter2/1
  Kalman Filter2/1 -> Gain6/1
  [VVMC_AvgRawWhlSpeed_kph] -> Gain8/1
  Gain8/1 -> Switch1/1
  VINP_GPSLAT_sec/1 -> Data Type Conversion1/1
  VINP_GPSLONG_sec/1 -> Data Type Conversion2/1
  Data Type Conversion1/1 -> [VINP_GPSLAT_sec]
  Data Type Conversion2/1 -> [VINP_GPSLONG_sec]
  Constant15/1 -> Delay/2
  Constant16/1 -> Delay1/2
  Gain1/1 -> Delay1/1, [VVMC_GPSLONG_rad]
  Constant17/1 -> Switch3/2
  [VVMC_GPSEstSpeed2_kph] -> Display4/1
  Gain9/1 -> [VVMC_GPSEstSpeed2_kph]  "VVMC_GPSEstSpeed2_kph"
  Gain10/1 -> Switch3/3
  Switch3/1 -> Kalman Filter4/2
  [VVMC_GPSSpd_mps] -> Switch3/1
  [VINP_VehSpeed_kph] -> Gain10/1
  Kalman Filter4/1 -> Gain9/1
  Sum of Elements1/1 -> Product1/1
  [VINP_VehSpeed_kph] -> Tapped Delay2/1
  Product1/1 -> [VVMC_RollAvgVehSpeed_kph]
  Width1/1 -> Product1/2
  Tapped Delay2/1 -> Width1/1, Sum of Elements1/1
  [VVMC_RollAvgVehSpeed_kph] -> Divide11/3
  [VVMC_LongAcc4Whl_Gps] -> Divide11/1
  [VVMC_GPSSpd_mps] -> Divide11/2
  Divide11/1 -> Kalman Filter4/1
  [VVMC_GPSEstSpeed3_kph] -> Display5/1
  Gain11/1 -> [VVMC_GPSEstSpeed3_kph]  "VVMC_GPSEstSpeed3_kph"
  [VVMC_GPSSpd_mps] -> Switch4/1
  Gain14/1 -> Switch4/3
  [VINP_VehSpeed_kph] -> Gain14/1
  [VVMC_LongAcc4Whl_Gps] -> Kalman Filter5/1
  Constant18/1 -> Switch4/2
  Kalman Filter5/1 -> Gain11/1
  Switch4/1 -> Kalman Filter5/2
  From50/1 -> Scheduler/1(task_time_s)
  Scheduler/1(trig_KF_10s()) -> Goto31/1
  [VVMC_LongAcc_Gps] -> Switch/3
  Switch/1 -> [VVMC_LongAcc4Whl_Gps]  "VVMC_LongAcc_Gps"
  [VINP_LongAccel_Gps] -> Switch/1
  Constant3/1 -> Switch/2
  VVMC_LongAcc_Gps/1 -> [VVMC_LongAcc_Gps]
  [VVMC_GPSSpd_mps] -> Switch5/1
  [VINP_VehSpeed_kph] -> Gain12/1
  Constant20/1 -> Switch5/2
  [VVMC_GPSEstSpeed4_kph] -> Display6/1
  Gain13/1 -> [VVMC_GPSEstSpeed4_kph]  "VVMC_GPSEstSpeed4_kph"
  [VVMC_RollAvgVehSpeed_kph] -> Divide12/3
  Switch5/1 -> Kalman Filter6/2
  [VVMC_GPSSpd_mps] -> Divide12/2
  Divide12/1 -> Kalman Filter6/1
  Kalman Filter6/1 -> Gain13/1
  [VVMC_LongAcc_Gps] -> Divide12/1
  Gain12/1 -> Switch5/3

== system vmc/VMC/ACC_Function/ACC Control Allow Judgement ==
  task_time_s : Inport
  VTQD_ExternalTqAllow_flag : Inport  Port=2
  VTQD_ExtDoorAllow_flg : Inport  Port=3
  AND : Logic  AllPortsSameDT=off  OutDataTypeStr=boolean
  Constant : Constant  Value=KVMC_ExternalTqAllowTime_s
  Constant3 : Constant  Value=TRUE
  Constant4 : Constant  Value=FALSE
  NOT : Logic  Operator=NOT  AllPortsSameDT=off  OutDataTypeStr=boolean
  Relational Operator : RelationalOperator  OutDataTypeStr=boolean  RndMeth=Simplest
  Timer : hcu_lib/Basic_Blocks/Timer
  u2>0 : Switch  Criteria=u2 > Threshold
  VVMC_ACCCtrlAllow_flg : Outport
  wires:
  task_time_s/1 -> [task_time_s]
  Constant/1 -> Relational Operator/2, Timer/4
  VTQD_ExternalTqAllow_flag/1 -> [VTQD_ExternalTqAllow_flag]
  NOT/1 -> Timer/2
  u2>0/1 -> [VVMC_ACCCtrlAllow_flg]  "VVMC_ACCCtrlAllow_flg"
  Constant4/1 -> u2>0/3
  Constant3/1 -> u2>0/1
  Timer/1 -> Relational Operator/1
  Relational Operator/1 -> u2>0/2
  [task_time_s] -> Timer/3
  [VVMC_ACCCtrlAllow_flg] -> VVMC_ACCCtrlAllow_flg/1
  VTQD_ExtDoorAllow_flg/1 -> [VTQD_ExtDoorAllow_flg]
  AND/1 -> NOT/1, Timer/1
  [VTQD_ExternalTqAllow_flag] -> AND/1
  [VTQD_ExtDoorAllow_flg] -> AND/2

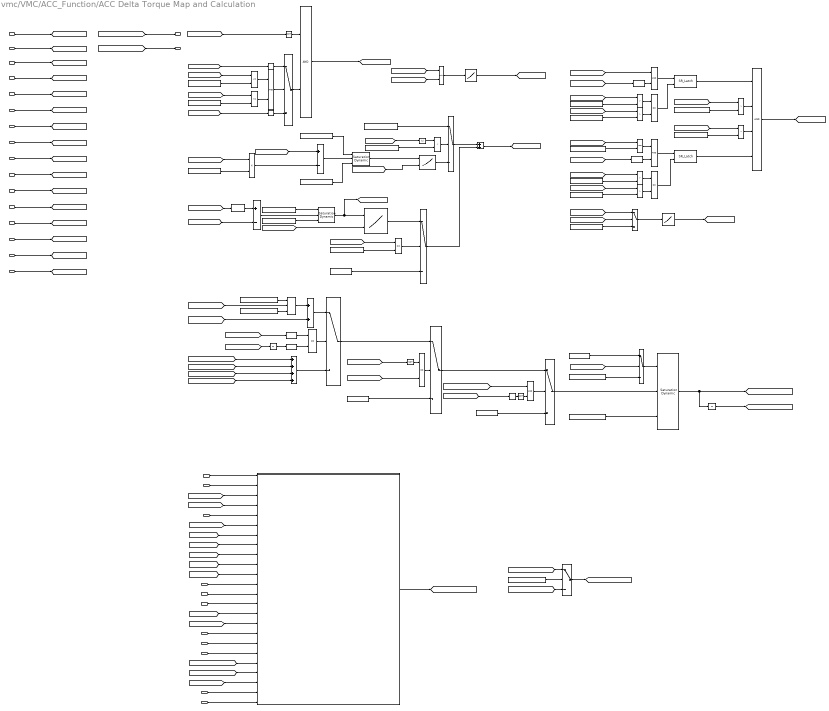
== system vmc/VMC/ACC_Function/ACC Delta Torque Map and Calculation ==
  VVMC_LongAcc_Gps : Inport
  VINP_ACCRequireAccel_mps2 : Inport  Port=2
  VINP_VehSpeed_kph : Inport  Port=3
  VTQD_DriverWhlTqDem_Nm : Inport  Port=4
  VVMC_ADASActive_flg : Inport  Port=5
  VVMC_ACCPedalOvrd_flg : Inport  Port=6
  VINP_ACCSetSpeed_enum : Inport  Port=7
  VINP_ACCVehHoldReq_flg : Inport  Port=8
  VINP_FrTMSpd_rpm : Inport  Port=9
  VINP_RrTMSpd_rpm : Inport  Port=10
  VINP_MCPressure_bar : Inport  Port=11
  VINP_ESCADASSta_enum : Inport  Port=12
  VINP_TargetType_enum : Inport  Port=13
  VVMC_CalMeterSpeed_kph : Inport  Port=14
  VINP_SWCResUpSta_flg : Inport  Port=15
  VVMC_EstSlope_Deg : Inport  Port=16
  VVMC_TotalAvailBrkRgnTq_Nm : Inport  Port=17
  VVMC_AccelTurnHold_flg : Inport  Port=18
  task_time_s : Inport  Port=19
  VVMC_TimeGapJudge_flag : Inport  Port=20
  VTQR_FrTMTqReq_Nm : Inport  Port=21
  VTQR_RrTMTqReq_Nm : Inport  Port=22
  VVMC_MeterIndSpeedForCalcu_kph : Inport  Port=23
  VINP_ADASACCSta_enum : Inport  Port=24
  VVMC_AfterCtrlACCReqAccel_mps2 : Inport  Port=25
  VVMC_ACCReqSpdMemory_kph : Inport  Port=26
  VVMC_ACCSpdCtrl_flg : Inport  Port=27
  AND{,2..4,7} (5 alike) : Logic  AllPortsSameDT=off  OutDataTypeStr=boolean
  AND1 : Logic  Inputs=4  AllPortsSameDT=off  OutDataTypeStr=boolean
  Abs : Abs
  Add : Sum
  Add1 : Sum  Inputs=+-
  Add2 : Sum  Inputs=++++
  Add3 : Sum
  Add5 : Sum  Inputs=+-
  Constant{,1,17,21,28} (5 alike) : Constant  Value=ZERO_FLOAT
  Constant10 : Constant  Value=KVMC_GravityValue_mps2
  Constant11 : Constant  Value=KVMC_AccDevLowLim_mps2
  Constant{9,12,15..16} (4 alike) : Constant  Value=KVMC_HillUpResetTMSpd_rpm
  Constant13 : Constant  Value=ENUM_ESCADASSTA_VEHASTANDSTILL
  Constant14 : Constant  Value=KVMC_ACCResUpEnAccCMD_mps2
  Constant18 : Constant  Value=ZERO_INT
  Constant19 : Constant  Value=KVMC_AccDevUpLim_mps2
  Constant2 : Constant  Value=KVMC_ADASWhlTqUpperLim_Nm
  Constant20 : Constant  Value=ENUM_TARGETTYPE_NONE
  Constant22 : Constant  Value=KVMC_NegReqSwEnSpd_kph
  Constant23 : Constant  Value=KVMC_ADASWheTqSWP2_flg
  Constant3 : Constant  Value=KVMC_ADASWhlTqLowerLim_Nm
  Constant32 : Constant  Value=KVMC_ACCResUpEnGrade_Deg
  Constant33 : Constant  Value=KVMC_ACCIGainOffDevSpd_kph
  Constant4 : Constant  Value=KVMC_ACCSpdDevUpLim_kph
  Constant5 : Constant  Value=KVMC_NegReqSwEnSlope_Deg
  Constant6 : Constant  Value=KVMC_ACCSpdDevLowLim_kph
  Constant7 : Constant  Value=KVMC_ACCPedal2TqUpLim_Nm
  Constant8 : Constant  Value=KVMC_ACCPedal2TqLowLim_Nm
  Data Type Conversion : DataTypeConversion  OutDataTypeStr=single
  Delay : Delay  DelayLength=1
  Detect Decrease1 : simulink/Logic and Bit Operations/Detect Decrease  vinit=0.0  OutDataTypeStr=boolean
  Detect Increase : simulink/Logic and Bit Operations/Detect Increase  vinit=0.0  OutDataTypeStr=boolean
  Detect Increase1 : simulink/Logic and Bit Operations/Detect Increase  vinit=0.0  OutDataTypeStr=boolean
  Detect Increase2 : simulink/Logic and Bit Operations/Detect Increase  vinit=0.0  OutDataTypeStr=boolean
  Equal : RelationalOperator  Operator===  OutDataTypeStr=boolean  RndMeth=Simplest
  Equal1 : RelationalOperator  Operator=<=  OutDataTypeStr=boolean  RndMeth=Simplest
  Equal2 : RelationalOperator  Operator===  OutDataTypeStr=boolean  RndMeth=Simplest
  Equal3 : RelationalOperator  OutDataTypeStr=boolean  RndMeth=Simplest
  InitialCondition: 0 : UnitDelay  SampleTime=-1  HasFrameUpgradeWarning=on
  Logical Operator : Logic  Operator=OR  AllPortsSameDT=off  OutDataTypeStr=boolean
  MVMC_ACCDeltaTqIGain_Z_Nm : Lookup_n-D  BreakpointsForDimension1=AVMC_ACCDeltaTqIGain_Y_mps2  BreakpointsForDimension2=AVMC_ACCDeltaTqIGain_X_kph  Table=MVMC_ACCDeltaTqIGain_Z_Nm  ExtrapMethod=Clip  InternalRulePriority=Speed  RndMeth=Simplest  InputSameDT=on
      settings: InputPortMap=u0,u1
  MVMC_ACCDeltaTqPGain_Z_Nm : Lookup_n-D  BreakpointsForDimension1=AVMC_ACCDeltaTqPGain_Y_kph  BreakpointsForDimension2=AVMC_ACCDeltaTqPGain_X_kph  Table=MVMC_ACCDeltaTqPGain_Z_Nm  ExtrapMethod=Clip  InternalRulePriority=Speed  RndMeth=Simplest  InputSameDT=on
      settings: InputPortMap=u0,u1
  MVMC_MCPresBaseTq_Y_Nm : Lookup_n-D  NumberOfTableDimensions=1  BreakpointsForDimension1=AVMC_MCPresBaseTq_X_bar  Table=MVMC_MCPresBaseTq_Y_Nm  ExtrapMethod=Clip  InternalRulePriority=Speed  RndMeth=Simplest  InputSameDT=on
  MVMC_TMSpdBaseTq_Y_Nm : Lookup_n-D  NumberOfTableDimensions=1  BreakpointsForDimension1=AVMC_TMSpdBaseTq_X_rpm  Table=MVMC_TMSpdBaseTq_Y_Nm  ExtrapMethod=Clip  InternalRulePriority=Speed  RndMeth=Simplest  InputSameDT=on
  Min : MinMax  Inputs=2
  NOT : Logic  Operator=NOT  AllPortsSameDT=off  OutDataTypeStr=boolean
  NOT1 : Logic  Operator=NOT  AllPortsSameDT=off  OutDataTypeStr=boolean
  NOT2 : Logic  Operator=NOT  AllPortsSameDT=off  OutDataTypeStr=boolean
  OR : Logic  Operator=OR  AllPortsSameDT=off  OutDataTypeStr=boolean
  OR1 : Logic  Operator=OR  AllPortsSameDT=off  OutDataTypeStr=boolean
  OR3 : Logic  Operator=OR  AllPortsSameDT=off  OutDataTypeStr=boolean
  Phase2_ADASWhlTqCal : Subsystem
  Product : Product
  Relational Operator{,1,3..6} (6 alike) : RelationalOperator  Operator=>  OutDataTypeStr=boolean  RndMeth=Simplest
  Relational Operator8 : RelationalOperator  Operator=<  OutDataTypeStr=boolean  RndMeth=Simplest
  Relay : Relay  OnSwitchValue=KVMC_ACCTq2ZeroEnMCPress2_bar  OffSwitchValue=KVMC_ACCTq2ZeroDisMCPress2_bar  OutDataTypeStr=boolean
  Relay1 : Relay  OnSwitchValue=KVMC_ACCTq2ZeroEnMCPress_bar  OffSwitchValue=KVMC_ACCTq2ZeroDisMCPress_bar  OutDataTypeStr=boolean
  SR_Latch : hcu_lib/Basic_Blocks/SR_Latch
  SR_Latch1 : hcu_lib/Basic_Blocks/SR_Latch
  Saturation Dynamic{,1..3} (4 alike) : simulink/Discontinuities/Saturation Dynamic  OutMin=[]  OutMax=[]  OutDataTypeStr=Inherit: Same as second input  OutDataType=fixdt(1, 16)  OutScaling=2^-10  DoSatur=off
  Switch{,1..6,9,11} (9 alike) : Switch  Criteria=u2 > Threshold
  Unit Delay : UnitDelay  SampleTime=-1  HasFrameUpgradeWarning=on
  VVMC_ADASWhlTqCal_Nm : Outport
  VVMC_ADASNegReq_flg : Outport  Port=2
  wires:
  Constant19/1 -> Saturation Dynamic1/1
  Product/1 -> Add1/2
  Add1/1 -> Saturation Dynamic1/2
  [VINP_ACCRequireAccel_mps2] -> Add1/1
  Constant10/1 -> Product/2
  [VVMC_LongAcc_Gps] -> Product/1
  Constant11/1 -> Saturation Dynamic1/3
  VVMC_LongAcc_Gps/1 -> [VVMC_LongAcc_Gps]
  VINP_ACCRequireAccel_mps2/1 -> [VINP_ACCRequireAccel_mps2]
  VINP_VehSpeed_kph/1 -> [VINP_VehSpeed_kph]
  VTQD_DriverWhlTqDem_Nm/1 -> [VTQD_DriverWhlTqDem_Nm]
  VVMC_ADASActive_flg/1 -> [VVMC_ADASActive_flg]
  [VVMC_ADASWhlTqCal_Nm] -> VVMC_ADASWhlTqCal_Nm/1
  Constant/1 -> Switch1/3
  Saturation Dynamic2/1 -> InitialCondition: 0/1, [VVMC_ADASWhlTqCalP1_Nm]  "VVMC_ADASWhlTqCal_Nm"
  [VVMC_ADASActive_flg] -> Detect Increase/1
  [VVMC_ACCDeltaTq_Nm] -> Add3/2
  Add3/1 -> Switch2/1
  InitialCondition: 0/1 -> [VVMC_LastADASWhlTqCal_Nm]  "VVMC_LastADASWhlTqCal_Nm"
  Saturation Dynamic1/1 -> MVMC_ACCDeltaTqIGain_Z_Nm/1  "VVMC_ActAccDev_mps2"
  Logical Operator/1 -> Switch2/2
  Switch3/1 -> Switch1/1
  Switch2/1 -> Switch3/1
  Add2/1 -> Switch2/3
  [VINP_VehSpeed_kph] -> MVMC_ACCDeltaTqIGain_Z_Nm/2
  VVMC_ACCPedalOvrd_flg/1 -> [VVMC_ACCPedalOvrd_flg]
  [VVMC_ACCPedalOvrd_flg] -> Unit Delay/1
  Detect Decrease1/1 -> Logical Operator/2
  Detect Increase/1 -> Logical Operator/1
  Switch1/1 -> Saturation Dynamic2/2
  Unit Delay/1 -> Detect Decrease1/1
  VINP_ACCSetSpeed_enum/1 -> [VINP_ACCSetSpeed_enum]
  [VINP_ACCSetSpeed_enum] -> Data Type Conversion/1
  [VVMC_CalMeterSpeed_kph] -> Add5/2
  Saturation Dynamic3/1 -> [VVMC_ACCActSpdDev_kph], MVMC_ACCDeltaTqPGain_Z_Nm/1  "VVMC_ACCActSpdDev_kph"
  Add5/1 -> Saturation Dynamic3/2
  Constant4/1 -> Saturation Dynamic3/1
  Constant6/1 -> Saturation Dynamic3/3
  Add/1 -> [VVMC_ACCDeltaTq_Nm]  "VVMC_ACCDeltaTq_Nm"
  Data Type Conversion/1 -> Add5/1
  Constant8/1 -> Saturation Dynamic/3
  [VTQD_DriverWhlTqDem_Nm] -> Saturation Dynamic/2
  Constant7/1 -> Saturation Dynamic/1
  Saturation Dynamic/1 -> Add3/1
  [VINP_VehSpeed_kph] -> MVMC_ACCDeltaTqPGain_Z_Nm/2
  VINP_ACCVehHoldReq_flg/1 -> [VINP_ACCVehHoldReq_flg]
  Constant1/1 -> Switch3/3
  Equal/1 -> AND/1
  OR/1 -> SR_Latch/2
  Relational Operator1/1 -> OR/2
  [VVMC_MCPreBaseTqEn_flg] -> Switch/2
  AND1/1 -> [VVMC_MCPreBaseTqEn_flg]  "VVMC_MCPreBaseTqEn_flg"
  SR_Latch/1 -> AND1/1  "VVMC_ACCVehHoldEn_flg"
  OR1/1 -> SR_Latch1/2
  Relational Operator4/1 -> OR1/2
  Relational Operator3/1 -> OR1/1
  Constant16/1 -> Relational Operator3/2
  [VINP_FrTMSpd_rpm] -> Relational Operator/1
  [VINP_MCPressure_bar] -> Switch/1
  [VINP_RrTMSpd_rpm] -> Relational Operator4/1
  Constant13/1 -> Equal/2
  [VINP_FrTMSpd_rpm] -> Relational Operator3/1
  Constant15/1 -> Relational Operator4/2
  [VINP_ESCADASSta_enum] -> Equal/1
  Constant12/1 -> Relational Operator1/2
  [VINP_RrTMSpd_rpm] -> Relational Operator1/1
  Switch/1 -> MVMC_MCPresBaseTq_Y_Nm/1
  Relational Operator/1 -> OR/1
  AND/1 -> SR_Latch1/1
  MVMC_MCPresBaseTq_Y_Nm/1 -> [VVMC_MCPresBaseTq_Nm]  "VVMC_MCPresBaseTq_Nm"
  Constant9/1 -> Relational Operator/2
  Constant17/1 -> Switch/3
  [VINP_RrTMSpd_rpm] -> Min/2
  MVMC_TMSpdBaseTq_Y_Nm/1 -> [VVMC_TMSpdBaseTq_Nm]  "VVMC_TMSpdBaseTq_Nm"
  [VINP_FrTMSpd_rpm] -> Min/1
  Min/1 -> MVMC_TMSpdBaseTq_Y_Nm/1
  VINP_MCPressure_bar/1 -> [VINP_MCPressure_bar]
  VINP_ESCADASSta_enum/1 -> [VINP_ESCADASSta_enum]
  VINP_FrTMSpd_rpm/1 -> [VINP_FrTMSpd_rpm]
  VINP_RrTMSpd_rpm/1 -> [VINP_RrTMSpd_rpm]
  [VVMC_MCPresBaseTq_Nm] -> Add2/4
  [VVMC_ACCDeltaTq_Nm] -> Add2/2
  [VVMC_LastADASWhlTqCal_Nm] -> Add2/1
  [VVMC_TMSpdBaseTq_Nm] -> Add2/3
  Constant20/1 -> Equal2/2
  [VINP_TargetType_enum] -> Equal2/1
  Equal2/1 -> Switch5/2
  Constant21/1 -> Switch5/3
  Switch5/1 -> Add/2  "VVMC_ACCDeltaTqPGain_Nm"
  [VINP_SWCResUpSta_flg] -> Detect Increase2/1
  Detect Increase2/1 -> AND3/2
  [VINP_ACCVehHoldReq_flg] -> AND3/1
  AND3/1 -> SR_Latch/1
  Detect Increase1/1 -> AND/2
  [VINP_SWCResUpSta_flg] -> Detect Increase1/1
  VINP_SWCResUpSta_flg/1 -> [VINP_SWCResUpSta_flg]
  VINP_TargetType_enum/1 -> [VINP_TargetType_enum]
  VVMC_CalMeterSpeed_kph/1 -> [VVMC_CalMeterSpeed_kph]
  [VINP_ACCRequireAccel_mps2] -> Relational Operator5/1
  Constant14/1 -> Relational Operator5/2
  MVMC_ACCDeltaTqPGain_Z_Nm/1 -> Switch5/1
  [VVMC_ADASNegReq_flg] -> Switch9/2
  Constant28/1 -> Switch9/1
  Constant2/1 -> Switch9/3
  Switch9/1 -> Saturation Dynamic2/1
  Constant3/1 -> Saturation Dynamic2/3
  NOT/1 -> OR3/1
  [VINP_ACCVehHoldReq_flg] -> NOT/1
  [VVMC_MCPreBaseTqEn_flg] -> OR3/2
  OR3/1 -> Switch3/2
  [VVMC_ADASNegReq_flg] -> VVMC_ADASNegReq_flg/1
  Constant32/1 -> Relational Operator6/2
  [VVMC_EstSlope_Deg] -> Relational Operator6/1
  Relational Operator5/1 -> AND1/2
  Relational Operator6/1 -> AND1/3
  SR_Latch1/1 -> AND1/4  "VVMC_HillUpESCStaEn_flg"
  VVMC_EstSlope_Deg/1 -> [VVMC_EstSlope_Deg]
  [VVMC_EstSlope_Deg] -> Equal3/1
  AND2/1 -> [VVMC_ADASNegReq_flg]  "VVMC_ADASNegReq_flg"
  [VINP_VehSpeed_kph] -> Equal1/1
  Equal3/1 -> AND7/2
  [VINP_MCPressure_bar] -> Relay1/1
  Equal1/1 -> AND7/1
  Constant22/1 -> Equal1/2
  Constant5/1 -> Equal3/2
  [VVMC_MCPreBaseTqEn_flg] -> NOT2/1
  Relay/1 -> Switch6/1
  [VINP_MCPressure_bar] -> Relay/1
  NOT2/1 -> AND2/1
  Relay1/1 -> Switch6/3
  AND7/1 -> Switch6/2
  Switch6/1 -> AND2/2
  Relational Operator8/1 -> Switch11/2
  Abs/1 -> Relational Operator8/1
  Constant18/1 -> Switch11/1
  Constant33/1 -> Relational Operator8/2
  [VVMC_ACCActSpdDev_kph] -> Abs/1
  MVMC_ACCDeltaTqIGain_Z_Nm/1 -> Switch11/3
  Switch11/1 -> Add/1  "VVMC_ACCDeltaTqIGain_Nm"
  [VVMC_ACCPedalOvrd_flg] -> Delay/1
  Delay/1 -> NOT1/1
  NOT1/1 -> AND4/2
  [VVMC_ADASActive_flg] -> AND4/1
  AND4/1 -> Switch1/2
  VVMC_TotalAvailBrkRgnTq_Nm/1 -> Phase2_ADASWhlTqCal/1(VVMC_TotalAvailBrkRgnTq_Nm)
  VVMC_AccelTurnHold_flg/1 -> Phase2_ADASWhlTqCal/2(VVMC_AccelTurnHold_flg)
  [VVMC_ADASActive_flg] -> Phase2_ADASWhlTqCal/3(VVMC_ADASActive_flg)
  [VVMC_ACCPedalOvrd_flg] -> Phase2_ADASWhlTqCal/4(VVMC_ACCPedalOvrd_flg)
  task_time_s/1 -> Phase2_ADASWhlTqCal/5(task_time_s)
  [VINP_ESCADASSta_enum] -> Phase2_ADASWhlTqCal/6(VINP_ESCADASSta_enum)
  [VVMC_MCPreBaseTqEn_flg] -> Phase2_ADASWhlTqCal/7(VVMC_MCPreBaseTqEn_flg)
  [VINP_ACCVehHoldReq_flg] -> Phase2_ADASWhlTqCal/8(VINP_ACCVehHoldReq_flg)
  [VINP_VehSpeed_kph] -> Phase2_ADASWhlTqCal/9(VINP_VehSpeed_kph)
  [VINP_MCPressure_bar] -> Phase2_ADASWhlTqCal/10(VINP_MCPressure_bar)
  [VVMC_ADASNegReq_flg] -> Phase2_ADASWhlTqCal/11(VVMC_ADASNegReq_flg)
  VVMC_TimeGapJudge_flag/1 -> Phase2_ADASWhlTqCal/12(VVMC_TimeGapJudge_flag)
  VTQR_FrTMTqReq_Nm/1 -> Phase2_ADASWhlTqCal/13(VTQR_FrTMTqReq_Nm)
  VTQR_RrTMTqReq_Nm/1 -> Phase2_ADASWhlTqCal/14(VTQR_RrTMTqReq_Nm)
  [VVMC_LongAcc_Gps] -> Phase2_ADASWhlTqCal/15(VVMC_LongAcc_Gps)
  [VINP_ACCSetSpeed_enum] -> Phase2_ADASWhlTqCal/16(VVMC_FeatSetSpdForCalcu_kph)
  VVMC_MeterIndSpeedForCalcu_kph/1 -> Phase2_ADASWhlTqCal/17(VVMC_MeterIndSpeedForCalcu_kph)
  Phase2_ADASWhlTqCal/1(VVMC_ADASWhlTqCal_Nm) -> [VVMC_ADASWhlTqCalP2_Nm]
  [VVMC_ADASWhlTqCalP1_Nm] -> Switch4/3
  [VVMC_ADASWhlTqCalP2_Nm] -> Switch4/1
  Constant23/1 -> Switch4/2
  Switch4/1 -> [VVMC_ADASWhlTqCal_Nm]
  VINP_ADASACCSta_enum/1 -> Phase2_ADASWhlTqCal/18(VINP_ADASACCSta_enum)
  VVMC_AfterCtrlACCReqAccel_mps2/1 -> Phase2_ADASWhlTqCal/19(VVMC_AfterCtrlACCReqAccel_mps2)
  [VVMC_TMSpdBaseTq_Nm] -> Phase2_ADASWhlTqCal/20(VVMC_TMSpdBaseTq_Nm)
  [VVMC_MCPresBaseTq_Nm] -> Phase2_ADASWhlTqCal/21(VVMC_MCPresBaseTq_Nm)
  [VVMC_EstSlope_Deg] -> Phase2_ADASWhlTqCal/22(VVMC_EstSlope_Deg)
  VVMC_ACCReqSpdMemory_kph/1 -> Phase2_ADASWhlTqCal/23(VVMC_ACCReqSpdMemory_kph)
  VVMC_ACCSpdCtrl_flg/1 -> Phase2_ADASWhlTqCal/24(VVMC_ACCSpdCtrl_flg)
